simulink model "UserOneButtonInputInterface"  (R2019b)
settings: Solver=FixedStepAuto  StartTime=0.0  StopTime=10.0  RelTol=1e-3
model workspace (MAT data in the model file):
  ADCResolution_C = Simulink.Parameter
  ADCResolution_C.Value = 4096
  ADCResolution_C.DataType = 'uint16'
  ADCResolution_C.DocUnits = 'b'
  ADCResolution_C.Dimensions = [1 1]
  PWMPeriod_D = Simulink.Parameter
  PWMPeriod_D.Value = 327
  PWMPeriod_D.DataType = 'single'
  PWMPeriod_D.Dimensions = [1 1]
libraries: simulink x2
settings Model: DataDictionary=UserOneButtonInterface.sldd  OrderedModelArguments=off  Creator=unix  LastModifiedBy=unix

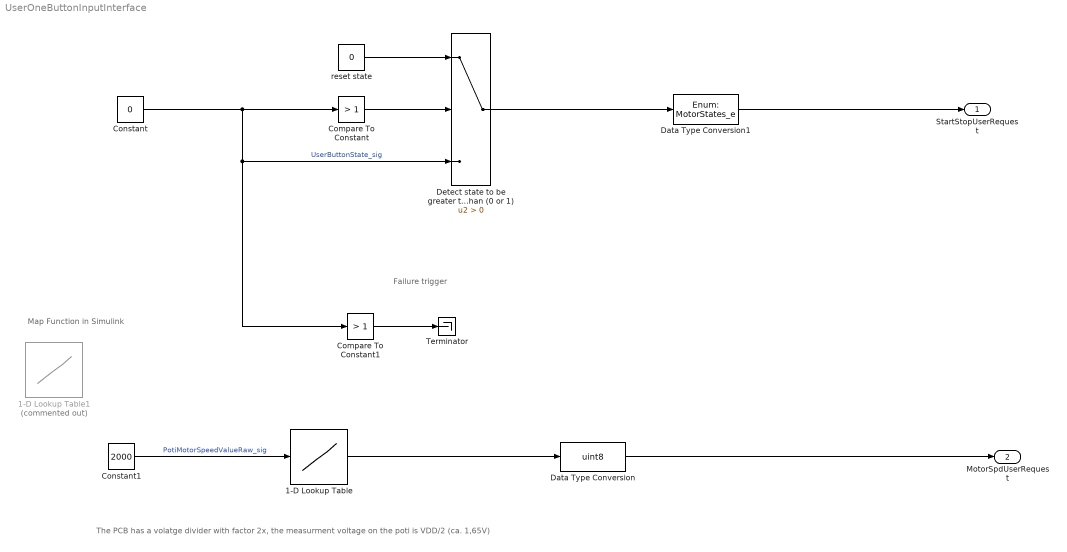
== system UserOneButtonInputInterface ==
  note: Map Function in Simulink
  note: The PCB has a volatge divider with factor 2x, the measurment voltage on the poti is VDD/2 (ca. 1,65V)
  note: Failure trigger
  1-D Lookup Table : Lookup_n-D  NumberOfTableDimensions=1  BreakpointsForDimension1=[0 (ADCResolution_C)/2]  Table=[0 100]  ExtrapMethod=Clip  InternalRulePriority=Speed  OutDataTypeStr=single  RndMeth=Simplest  InputSameDT=on
  1-D Lookup Table1 : Lookup_n-D  Commented=on  NumberOfTableDimensions=1  BreakpointsForDimension1=[0 (ADCResolution_C)/2]  Table=[0 PWMPeriod_D]  ExtrapMethod=Clip  InternalRulePriority=Speed  OutDataTypeStr=Inherit: Inherit from 'Table data'  RndMeth=Simplest  InputSameDT=on
  Compare To Constant : simulink/Logic and Bit Operations/Compare To Constant  relop=>  const=1  OutDataTypeStr=boolean
  Compare To Constant1 : simulink/Logic and Bit Operations/Compare To Constant  relop=>  const=1  OutDataTypeStr=boolean
  Constant : Constant  Value=0  OutDataTypeStr=Inherit: Inherit via back propagation
  Constant1 : Constant  Value=2000  OutDataTypeStr=Inherit: Inherit via back propagation
  Data Type Conversion : DataTypeConversion  OutDataTypeStr=uint8  RndMeth=Nearest
  Data Type Conversion1 : DataTypeConversion  OutDataTypeStr=Enum: MotorStates_e
  Detect state to be greater than (0 or 1) : Switch  Criteria=u2 > Threshold
  Terminator : Terminator
  reset state : Constant  Value=0  OutDataTypeStr=boolean
  StartStopUserRequest : Outport
  MotorSpdUserRequest : Outport  Port=2
  wires:
  Constant/1 -> Compare To Constant1/1, Detect state to be greater than (0 or 1)/3, Compare To Constant/1  "UserButtonState_sig"
  Compare To Constant/1 -> Detect state to be greater than (0 or 1)/2
  reset state/1 -> Detect state to be greater than (0 or 1)/1
  Detect state to be greater than (0 or 1)/1 -> Data Type Conversion1/1
  Constant1/1 -> 1-D Lookup Table/1  "PotiMotorSpeedValueRaw_sig"
  1-D Lookup Table/1 -> Data Type Conversion/1
  Compare To Constant1/1 -> Terminator/1
  Data Type Conversion/1 -> MotorSpdUserRequest/1
  Data Type Conversion1/1 -> StartStopUserRequest/1
